simulink model "identification_moteur"  (R2016b)
settings: Solver=VariableStepAuto  StartTime=0.0  StopTime=14  RelTol=1e-3
values from neighbouring files (symbols this model uses):
  Km = (4900-2250)/(4780-4416)    (= 7.28021978022)    [conv_fichier_bo.m]
  Tm = 0.15    [conv_fichier_bo.m]
settings Model: Creator=emiliendurif  LastModifiedBy=emiliendurif

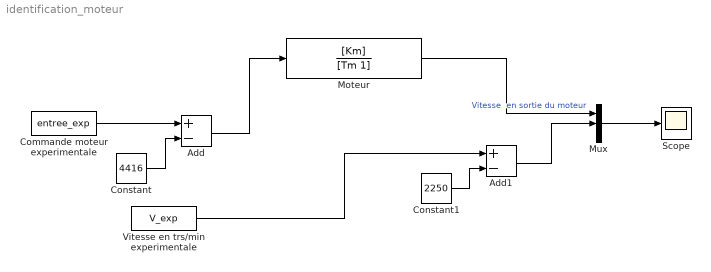
== system identification_moteur ==
  Add : Sum  Inputs=+-
  Add1 : Sum  Inputs=+-
  Commande moteur experimentale : FromWorkspace  VariableName=entree_exp  OutDataTypeStr=fixdt('double', 'DataTypeOverride', 'Off')  SampleTime=0.007  OutputAfterFinalValue=Setting to zero
  Constant : Constant  Value=4416
  Constant1 : Constant  Value=2250
  "Moteur " : TransferFcn  Numerator=[Km]  Denominator=[Tm 1]
  Mux : Mux  Inputs=3
  Scope : Scope
  Vitesse en trs/min experimentale : FromWorkspace  VariableName=V_exp  OutDataTypeStr=fixdt('double', 'DataTypeOverride', 'Off')  SampleTime=0.007  OutputAfterFinalValue=Setting to zero
  wires:
  Constant/1 -> Add/2
  "Moteur "/1 -> Mux/1  "Vitesse  en sortie du moteur"
  Mux/1 -> Scope/1
  Commande moteur experimentale/1 -> Add/1
  Add/1 -> "Moteur "/1
  Vitesse en trs/min experimentale/1 -> Add1/1
  Constant1/1 -> Add1/2
  Add1/1 -> Mux/2
